simulink model "PMDC_controller"  (R2023a)
settings: Solver=VariableStepAuto  StartTime=0.0  StopTime=10.0  RelTol=1e-3
values from neighbouring files (symbols this model uses):
  Gc = 1/(Ri+s*Li)    [PMDC_par.m]
  Gw = 1/(beta+s*J)    [PMDC_par.m]
  K = 0.04    [PMDC_par.m]
  Rc = kp+ki/s    [PMDC_par.m]
  Rw = wc_w*beta/s*(1+s/166.7)    [PMDC_par.m]
  w_ref = 300    [PMDC_par.m]
settings Model: Creator=Andrea  LastModifiedBy=Andrea
settings OptimizationCC: ReuseModelBlockBuffer=off

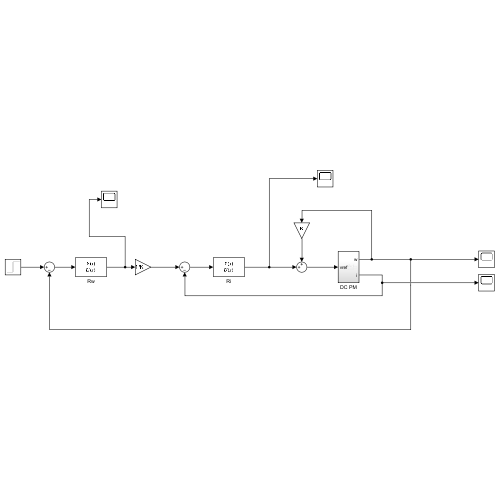
[thumbnail: Simulink's stored preview of the top-level diagram]
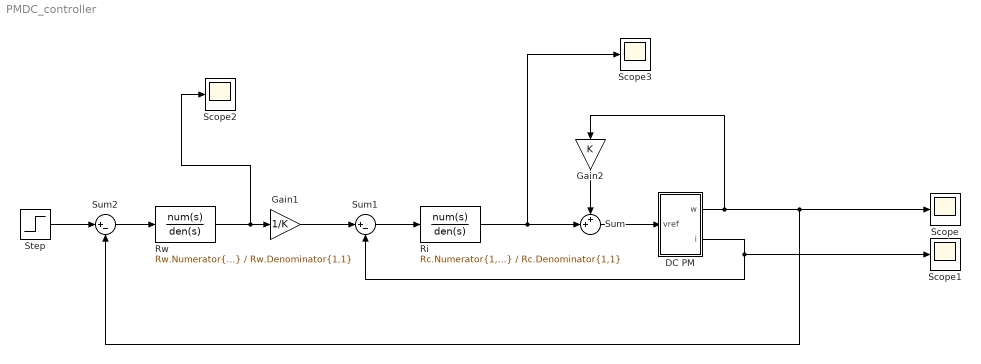
== system PMDC_controller ==
  DC PM : Subsystem
  Gain1 : Gain  Gain=1/K
  Gain2 : Gain  Gain=K
  Ri : TransferFcn  Numerator=Rc.Numerator{1,1}  Denominator=Rc.Denominator{1,1}
  Rw : TransferFcn  Numerator=Rw.Numerator{1,1}  Denominator=Rw.Denominator{1,1}
  Scope{,1..3} (4 alike) : Scope
  Step : Step  Time=0  After=w_ref  SampleTime=0
  Sum : Sum  Inputs=++|
  Sum1 : Sum  Inputs=|+-
  Sum2 : Sum  Inputs=|+-
  wires:
  DC PM/1(w) -> Sum2/2, Scope/1, Gain2/1
  Sum/1 -> DC PM/1(vref)
  Sum1/1 -> Ri/1
  Rw/1 -> Scope2/1, Gain1/1
  Sum2/1 -> Rw/1
  Step/1 -> Sum2/1
  Gain2/1 -> Sum/1
  DC PM/2(i) -> Sum1/2, Scope1/1
  Gain1/1 -> Sum1/1
  Ri/1 -> Sum/2, Scope3/1

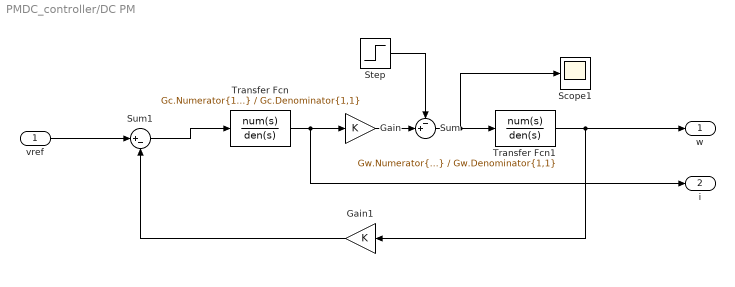
== system PMDC_controller/DC PM ==
  vref : Inport
  Gain : Gain  Gain=K
  Gain1 : Gain  Gain=K
  Scope1 : Scope
  Step : Step  Time=0.05  After=3  SampleTime=0
  Sum : Sum  Inputs=-+|
  Sum1 : Sum  Inputs=|+-
  Transfer Fcn : TransferFcn  Numerator=Gc.Numerator{1,1}  Denominator=Gc.Denominator{1,1}
  Transfer Fcn1 : TransferFcn  Numerator=Gw.Numerator{1,1}  Denominator=Gw.Denominator{1,1}
  w : Outport
  i : Outport  Port=2
  wires:
  Sum/1 -> Scope1/1, Transfer Fcn1/1
  Sum1/1 -> Transfer Fcn/1
  Transfer Fcn1/1 -> w/1, Gain1/1
  Gain/1 -> Sum/2
  Transfer Fcn/1 -> i/1, Gain/1
  Step/1 -> Sum/1
  vref/1 -> Sum1/1
  Gain1/1 -> Sum1/2
